simulink model "sim_mdl_iterative"  (R2020a)
settings: Solver=FixedStepAuto  StartTime=0.0  StopTime=1  FixedStep=0.001  RelTol=1e-8  AbsTol=1e-8  EnableMultiTasking=on
PreLoadFcn:
  | i=k;
values from neighbouring files (symbols this model uses):
  k = k'    [main_iterative.m]    (also in norm_range_solve.m = 1)
settings Model: Creator=Administrator  LastModifiedBy=78253
settings SolverCC: AutoScaleAbsTol=off  ZeroCrossAlgorithm=Non-adaptive
settings DataIOCC: LimitDataPoints=on  MaxDataPoints=10000  SaveFormat=Array  SignalLoggingSaveFormat=ModelDataLogs  ReturnWorkspaceOutputs=off  SignalLoggingName=sigsOut
settings OptimizationCC: ExpressionDepthLimit=2147483647  InitFltsAndDblsToZero=on  LifeSpan=inf
settings DebuggingCC: SaveWithParameterizedLinksMsg=none  UnderspecifiedInitializationDetection=Classic  MergeDetectMultiDrivingBlocksExec=none  SignalResolutionControl=TryResolveAllWithWarning  MultiTaskDSMMsg=warning  MultiTaskCondExecSysMsg=none  FcnCallInpInsideContextMsg=warning  StateNameClashWarn=warning  SFUnexpectedBacktrackingDiag=warning  SFNoUnconditionalDefaultTransitionDiag=warning  SFExecutionAtInitializationDiag=none  ArithmeticOperatorsInVariantConditions=warning
settings HardwareCC: ProdBitPerPointer=32  ProdBitPerSizeT=32  ProdBitPerPtrDiffT=32  ProdLargestAtomicFloat=None  ProdIntDivRoundTo=Undefined  ProdEndianess=Unspecified  ProdWordSize=32  ProdHWDeviceType=32-bit Generic  TargetUnknown=on
settings ModelReferenceCC: PropagateSignalLabelsOutOfModel=off
settings CodeAppCC: StateflowObjectComments=on
settings GRTTargetCC: TargetLangStandard=C89/C90 (ANSI)  CombineOutputUpdateFcns=off  GRTInterface=on
settings ConfigComp: CovMetricSettings=dw  CovHtmlReporting=on  CovSaveCumulativeToWorkspaceVar=on  CovSaveSingleToWorkspaceVar=on

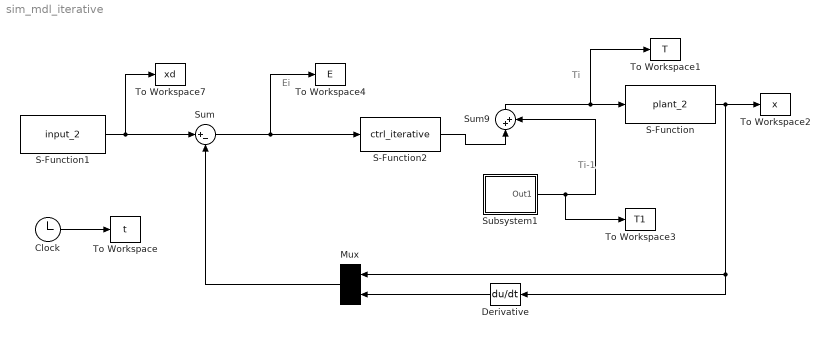
== system sim_mdl_iterative ==
  note: Ei
  note: Ti-1
  note: Ti
  Clock : Clock
  Derivative : Derivative
  Mux : Mux  Inputs=2
  S-Function : S-Function  FunctionName=plant_2  SFunctionDeploymentMode=off  EnableBusSupport=off
  S-Function1 : S-Function  FunctionName=input_2  SFunctionDeploymentMode=off  EnableBusSupport=off
  S-Function2 : S-Function  FunctionName=ctrl_iterative  SFunctionDeploymentMode=off  EnableBusSupport=off
  Subsystem1 : Subsystem
  Sum : Sum  Inputs=|+-  SaturateOnIntegerOverflow=on
  Sum9 : Sum  Inputs=|++  SaturateOnIntegerOverflow=on
  To Workspace : ToWorkspace  VariableName=t  SampleTime=-1
  To Workspace1 : ToWorkspace  VariableName=T  SampleTime=-1
  To Workspace2 : ToWorkspace  VariableName=x  SampleTime=-1
  To Workspace3 : ToWorkspace  VariableName=T1  SampleTime=-1
  To Workspace4 : ToWorkspace  VariableName=E  SampleTime=-1
  To Workspace7 : ToWorkspace  VariableName=xd  SampleTime=-1
  wires:
  Clock/1 -> To Workspace/1
  S-Function1/1 -> To Workspace7/1, Sum/1
  S-Function/1 -> To Workspace2/1, Derivative/1, Mux/1
  S-Function2/1 -> Sum9/1
  Sum9/1 -> S-Function/1, To Workspace1/1
  Sum/1 -> To Workspace4/1, S-Function2/1
  Mux/1 -> Sum/2
  Derivative/1 -> Mux/2
  Subsystem1/1(Out1) -> Sum9/2, To Workspace3/1

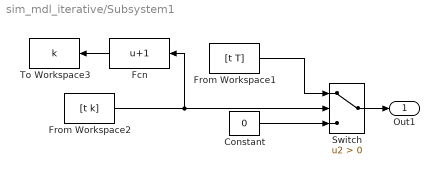
== system sim_mdl_iterative/Subsystem1 ==
  Constant : Constant  Value=0
  Fcn : Fcn  Expr=u+1
  From Workspace1 : FromWorkspace  VariableName=[t T]  ZeroCross=off
  From Workspace2 : FromWorkspace  VariableName=[t k]  ZeroCross=off
  Switch : Switch  Criteria=u2 > Threshold  SaturateOnIntegerOverflow=on
  To Workspace3 : ToWorkspace  VariableName=k  SampleTime=-1
  Out1 : Outport
  wires:
  Constant/1 -> Switch/3
  From Workspace1/1 -> Switch/1
  From Workspace2/1 -> Fcn/1, Switch/2
  Fcn/1 -> To Workspace3/1
  Switch/1 -> Out1/1
